simulink library "lduc_lib"  (Simulink 8.7)
settings: Solver=ode45  StartTime=0.0  StopTime=10.0  RelTol=1e-3
undefined symbols (not defined in the file): display, DUC_LINEUP_param, value
libraries: DSPBAFilters x6, DSPBAPrim x6, DSPBABase x6
settings Model: Creator=bigcat  LastModifiedBy=5g

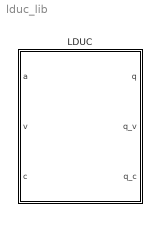
== system lduc_lib ==
  LDUC : Subsystem  mask{Clock_Margin=DUC_LINEUP_param.ClockMargin, chan_filter_SampleRate=DUC_LINEUP_param.chan_filter.SampleRate, chan_filter_ChanCount=DUC_LINEUP_param.chan_filter.ChanCount, chan_filter_coeffs=DUC_LINEUP_param.chan_filter.coeffs(1,:), chan_filter_base_addr=DUC_LINEUP_param.chan_filter.base_addr1, HB_filt4_SampleRate=DUC_LINEUP_param.HB_filt4.SampleRate, HB_filt_Interpolation=DUC_LINEUP_param.HB_filt4.Interpolation, HB_filt4_ChanCount=DUC_LINEUP_param.HB_filt4.ChanCount, HB_filt4_coeffs=DUC_LINEUP_param.HB_filt4.coeffs(1,:), HB_filt4_base_addr=DUC_LINEUP_param.HB_filt4.base_addr1, HB_filt5_SampleRate=DUC_LINEUP_param.HB_filt5.SampleRate, HB_filt5_Interpolation=DUC_LINEUP_param.HB_filt5.Interpolation, HB_filt5_ChanCount=DUC_LINEUP_param.HB_filt5.ChanCount, HB_filt5_coeffs=DUC_LINEUP_param.HB_filt5.coeffs(1,:), HB_filt5_base_addr=DUC_LINEUP_param.HB_filt5.base_addr1, Pipe_Reg=2, CH_Multiplication_fact=1, CH_Bits_to_Left_shift=0, HB4_Multiplication_fact=1, HB4_Bits_to_left_shift=1, HB5_Multiplication_fact=1, HB5_Bits_to_Left_shift=1, output_word_length=DUC_LINEUP_param.output_word_length, output_fraction_length=DUC_LINEUP_param.output_fraction_length}
      mask Display:
      | disp('LDUC');
      | port_label('input',1,'d');
      | port_label('input',2,'v');
      | port_label('input',3,'c');
      | port_label('output',1,'q');
      | port_label('output',2,'qv');
      | port_label('output',3,'qc');

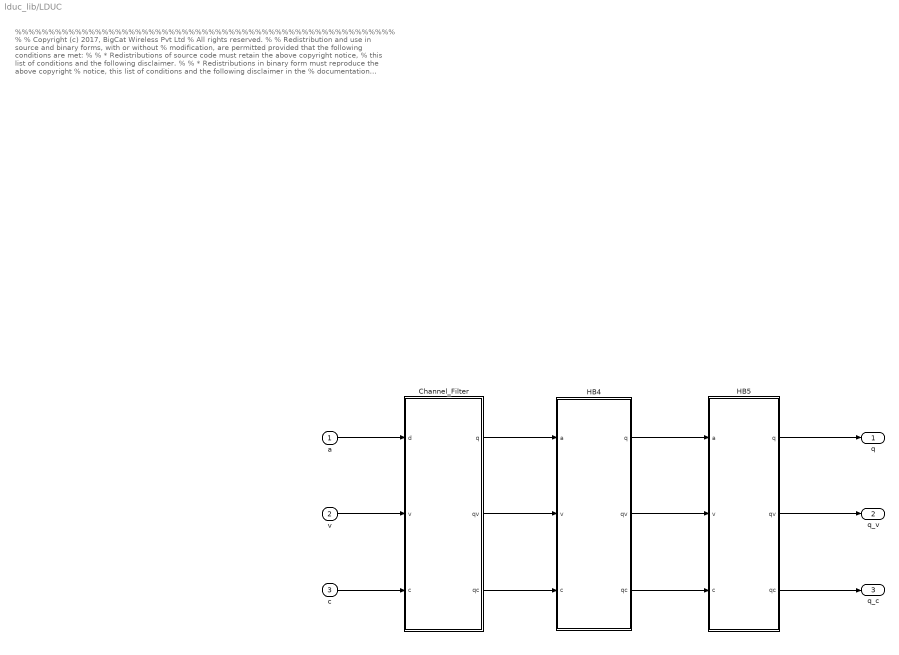
== system lduc_lib/LDUC ==
  note: %%%%%%%%%%%%%%%%%%%%%%%%%%%%%%%%%%%%%%%%%%%%%%%%%%%%%%%%%
      |  %
      |  % Copyright (c) 2017, BigCat Wireless Pvt Ltd
      |  % All rights reserved.
      |  %
      |  % Redistribution and use in source and binary forms, with or without
      |  % modification, are permitted provided that the following conditions are met:
      |  %
      |  %     * Redistributions of source code must retain the above copyright notice,
      |  %       this list of conditions and the following disclaimer.
      |  %
      |  %     * Redistributions in binary form must reproduce the above copyright
      |  %       notice, this list of conditions and the following disclaimer in the
      |  %       documentation and/or other materials provided with the distribution.
      |  %
      |  %     * Neither the name of the copyright holder nor the names of its contributors
      |  %       may be used to endorse or promote products derived from this software
      |  %       without specific prior written permission.
      |  %
      |  %
      |  %
      |  % THIS SOFTWARE IS PROVIDED BY THE COPYRIGHT HOLDERS AND CONTRIBUTORS "AS IS"
      |  % AND ANY EXPRESS OR IMPLIED WARRANTIES, INCLUDING, BUT NOT LIMITED TO, THE
      |  % IMPLIED WARRANTIES OF MERCHANTABILITY AND FITNESS FOR A PARTICULAR PURPOSE ARE
      |  % DISCLAIMED. IN NO EVENT SHALL THE COPYRIGHT HOLDER OR CONTRIBUTORS BE LIABLE
      |  % FOR ANY DIRECT, INDIRECT, INCIDENTAL, SPECIAL, EXEMPLARY, OR CONSEQUENTIAL
      |  % DAMAGES (INCLUDING, BUT NOT LIMITED TO, PROCUREMENT OF SUBSTITUTE GOODS OR
      |  % SERVICES; LOSS OF USE, DATA, OR PROFITS; OR BUSINESS INTERRUPTION) HOWEVER
      |  % CAUSED AND ON ANY THEORY OF LIABILITY, WHETHER IN CONTRACT, STRICT LIABILITY,
      |  % OR TORT (INCLUDING NEGLIGENCE OR OTHERWISE) ARISING IN ANY WAY OUT OF THE USE
      |  % OF THIS SOFTWARE, EVEN IF ADVISED OF THE POSSIBILITY OF SUCH DAMAGE.
      |  %
      |   %%%%%%%%%%%%%%%%%%%%%%%%%%%%%%%%%%%%%%%%%%%%%%%%%%%%%%%%%%
  a : Inport
  v : Inport  Port=2
  c : Inport  Port=3
  Channel_Filter : Subsystem
  HB4 : Subsystem
  HB5 : Subsystem
  q : Outport
  q_v : Outport  Port=2
  q_c : Outport  Port=3
  wires:
  Channel_Filter/3(qc) -> HB4/3(c)
  Channel_Filter/2(qv) -> HB4/2(v)
  Channel_Filter/1(q) -> HB4/1(a)
  a/1 -> Channel_Filter/1(d)
  v/1 -> Channel_Filter/2(v)
  c/1 -> Channel_Filter/3(c)
  HB5/1(q) -> q/1
  HB5/2(qv) -> q_v/1
  HB5/3(qc) -> q_c/1
  HB4/2(qv) -> HB5/2(v)
  HB4/1(q) -> HB5/1(a)
  HB4/3(qc) -> HB5/3(c)

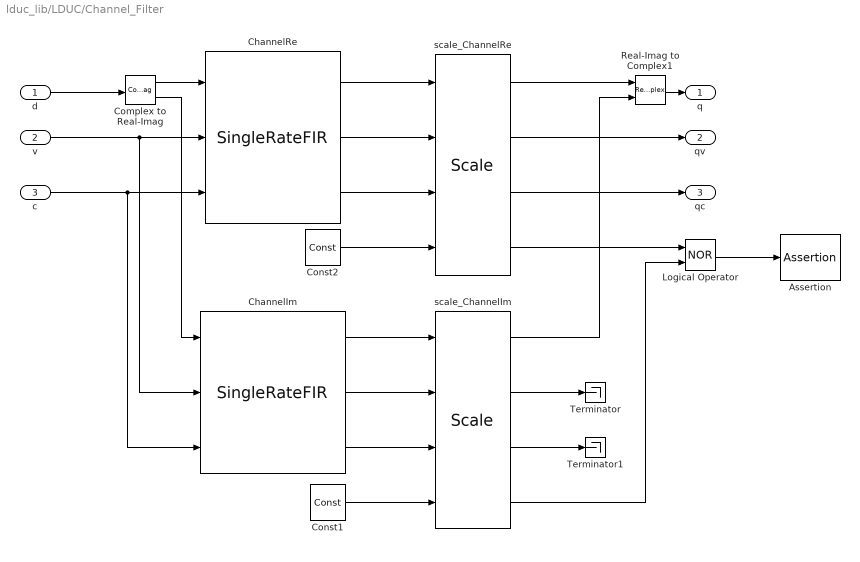
== system lduc_lib/LDUC/Channel_Filter ==
  d : Inport
  v : Inport  Port=2
  c : Inport  Port=3
  Assertion : Assertion  Enabled=off  AssertionFailFcn=display('Simulation stopped because of over/underflow in channel filter in LDUC')
  ChannelIm : DSPBAFilters/SingleRateFIR  nInputRate=chan_filter_SampleRate  nchan=chan_filter_ChanCount/2  symmetry=Symmetrical  coef=chan_filter_coeffs(1,:)  addr=chan_filter_base_addr+128  rwmode=Read/Write  nband=Use All Taps  latency=4  exposebus=off  version=20090407  recon=off  MM=[0,1,2,3,4,5,6,7,8,9,10,11,12,13,14,15;0,1,2,3,4,5,6,7,8,9,10,11,12,13,14,15]
  ChannelRe : DSPBAFilters/SingleRateFIR  nInputRate=chan_filter_SampleRate  nchan=chan_filter_ChanCount/2  symmetry=Symmetrical  coef=chan_filter_coeffs(1,:)  addr=chan_filter_base_addr  rwmode=Read/Write  nband=Use All Taps  latency=4  exposebus=off  version=20090407  recon=off  MM=[0,1,2,3,4,5,6,7,8,9,10,11,12,13,14,15;0,1,2,3,4,5,6,7,8,9,10,11,12,13,14,15]
  Complex to Real-Imag : ComplexToRealImag
  Const1 : DSPBAPrim/Const  primtype=const  nInputs=0  nOutputs=1  omode=Inherit via internal rule  otype=sfix(16)  scale=2^-15  rndmethod=Unbiased  factor=1  satmethod=Symmetric  shift_vec=[0 1 2 -1]  value=0  inPortNames=['+'; '+';]  outPortNames=[' ']  dspbaimage=dspba_prim.jpg  text=fprintf('%s', num2str(value));  style=Optimised  visibilities=8 + 1024  floatPrecision=float32_m23  version=20120820
  Const2 : DSPBAPrim/Const  primtype=const  nInputs=0  nOutputs=1  omode=Inherit via internal rule  otype=sfix(16)  scale=2^-15  rndmethod=Unbiased  factor=1  satmethod=Symmetric  shift_vec=[0 1 2 -1]  value=0  inPortNames=['+'; '+';]  outPortNames=[' ']  dspbaimage=dspba_prim.jpg  text=fprintf('%s', num2str(value));  style=Optimised  visibilities=8 + 1024  floatPrecision=float32_m23  version=20120820
  Logical Operator : Logic  Operator=NOR  AllPortsSameDT=off  OutDataTypeStr=boolean
  Real-Imag to Complex1 : RealImagToComplex
  Terminator : Terminator
  Terminator1 : Terminator
  scale_ChannelIm : DSPBABase/Scale  otype=sfix(output_word_length)  scale=2^-output_fraction_length  rndmethod=Truncate  factor=CH_Multiplication_fact  satmethod=Symmetric  shift_vec=CH_Bits_to_Left_shift  latency=4  wideSimulation=off  version=20090407
  scale_ChannelRe : DSPBABase/Scale  otype=sfix(output_word_length)  scale=2^-output_fraction_length  rndmethod=Truncate  factor=CH_Multiplication_fact  satmethod=Symmetric  shift_vec=CH_Bits_to_Left_shift  latency=4  wideSimulation=off  version=20090407
  q : Outport
  qv : Outport  Port=2
  qc : Outport  Port=3
  wires:
  Logical Operator/1 -> Assertion/1
  scale_ChannelIm/4 -> Logical Operator/2
  scale_ChannelIm/3 -> Terminator1/1
  scale_ChannelIm/2 -> Terminator/1
  scale_ChannelIm/1 -> Real-Imag to Complex1/2
  ChannelIm/3 -> scale_ChannelIm/3
  ChannelIm/2 -> scale_ChannelIm/2
  ChannelIm/1 -> scale_ChannelIm/1
  Real-Imag to Complex1/1 -> q/1
  scale_ChannelRe/1 -> Real-Imag to Complex1/1
  Const1/1 -> scale_ChannelIm/4
  Complex to Real-Imag/2 -> ChannelIm/1
  Complex to Real-Imag/1 -> ChannelRe/1
  d/1 -> Complex to Real-Imag/1
  ChannelRe/1 -> scale_ChannelRe/1
  c/1 -> ChannelIm/3, ChannelRe/3
  v/1 -> ChannelIm/2, ChannelRe/2
  scale_ChannelRe/3 -> qc/1
  Const2/1 -> scale_ChannelRe/4
  scale_ChannelRe/2 -> qv/1
  ChannelRe/2 -> scale_ChannelRe/2
  ChannelRe/3 -> scale_ChannelRe/3
  scale_ChannelRe/4 -> Logical Operator/1

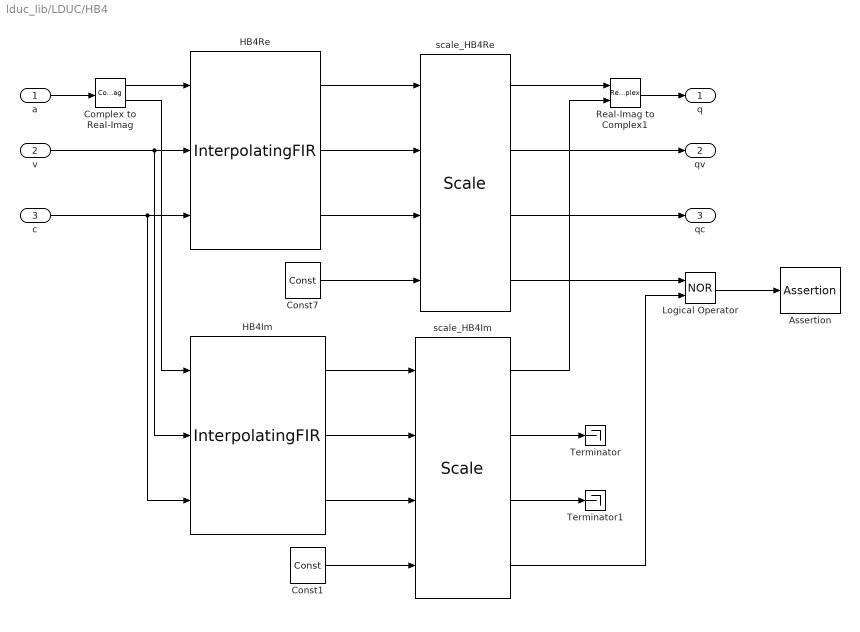
== system lduc_lib/LDUC/HB4 ==
  a : Inport
  v : Inport  Port=2
  c : Inport  Port=3
  Assertion : Assertion  Enabled=off  AssertionFailFcn=display('Simulation stopped because of over/underflow in HB4 filter in LDUC')
  Complex to Real-Imag : ComplexToRealImag
  Const1 : DSPBAPrim/Const  primtype=const  nInputs=0  nOutputs=1  omode=Inherit via internal rule  otype=sfix(16)  scale=2^-15  rndmethod=Unbiased  factor=1  satmethod=Symmetric  shift_vec=[0 1 2 -1]  value=0  inPortNames=['+'; '+';]  outPortNames=[' ']  dspbaimage=dspba_prim.jpg  text=fprintf('%s', num2str(value));  style=Optimised  visibilities=8 + 1024  floatPrecision=float32_m23  version=20120820
  Const7 : DSPBAPrim/Const  primtype=const  nInputs=0  nOutputs=1  omode=Inherit via internal rule  otype=sfix(16)  scale=2^-15  rndmethod=Unbiased  factor=1  satmethod=Symmetric  shift_vec=[0 1 2 -1]  value=0  inPortNames=['+'; '+';]  outPortNames=[' ']  dspbaimage=dspba_prim.jpg  text=fprintf('%s', num2str(value));  style=Optimised  visibilities=8 + 1024  floatPrecision=float32_m23  version=20120820
  HB4Im : DSPBAFilters/InterpolatingFIR  nInputRate=HB_filt4_SampleRate  interp=HB_filt_Interpolation  nchan=HB_filt4_ChanCount/2  symmetry=Symmetrical  coef=HB_filt4_coeffs(1,:)  addr=HB_filt4_base_addr+128  rwmode=Constant  nband=Half Band  exposebus=off  latency=14  version=20090407  recon=off  MM=[0,1,2,3,4,5,6,7,8,9,10,11,12,13,14,15]
  HB4Re : DSPBAFilters/InterpolatingFIR  nInputRate=HB_filt4_SampleRate  interp=HB_filt_Interpolation  nchan=HB_filt4_ChanCount/2  symmetry=Symmetrical  coef=HB_filt4_coeffs(1,:)  addr=HB_filt4_base_addr  rwmode=Constant  nband=Half Band  exposebus=off  latency=14  version=20090407  recon=off  MM=[0,1,2,3,4,5,6,7,8,9,10,11,12,13,14,15]
  Logical Operator : Logic  Operator=NOR  AllPortsSameDT=off  OutDataTypeStr=boolean
  Real-Imag to Complex1 : RealImagToComplex
  Terminator : Terminator
  Terminator1 : Terminator
  scale_HB4Im : DSPBABase/Scale  otype=sfix(output_word_length)  scale=2^-output_fraction_length  rndmethod=Truncate  factor=HB4_Multiplication_fact  satmethod=Symmetric  shift_vec=HB4_Bits_to_left_shift  latency=4  wideSimulation=off  version=20090407
  scale_HB4Re : DSPBABase/Scale  otype=sfix(output_word_length)  scale=2^-output_fraction_length  rndmethod=Truncate  factor=HB4_Multiplication_fact  satmethod=Symmetric  shift_vec=HB4_Bits_to_left_shift  latency=4  wideSimulation=off  version=20090407
  q : Outport
  qv : Outport  Port=2
  qc : Outport  Port=3
  wires:
  Logical Operator/1 -> Assertion/1
  scale_HB4Im/4 -> Logical Operator/2
  scale_HB4Im/3 -> Terminator1/1
  scale_HB4Im/2 -> Terminator/1
  Real-Imag to Complex1/1 -> q/1
  scale_HB4Im/1 -> Real-Imag to Complex1/2
  HB4Im/3 -> scale_HB4Im/3
  HB4Im/2 -> scale_HB4Im/2
  scale_HB4Re/1 -> Real-Imag to Complex1/1
  Const1/1 -> scale_HB4Im/4
  HB4Im/1 -> scale_HB4Im/1
  Complex to Real-Imag/2 -> HB4Im/1
  HB4Re/1 -> scale_HB4Re/1
  Complex to Real-Imag/1 -> HB4Re/1
  a/1 -> Complex to Real-Imag/1
  Const7/1 -> scale_HB4Re/4
  HB4Re/3 -> scale_HB4Re/3
  HB4Re/2 -> scale_HB4Re/2
  scale_HB4Re/3 -> qc/1
  scale_HB4Re/2 -> qv/1
  scale_HB4Re/4 -> Logical Operator/1
  c/1 -> HB4Im/3, HB4Re/3
  v/1 -> HB4Im/2, HB4Re/2

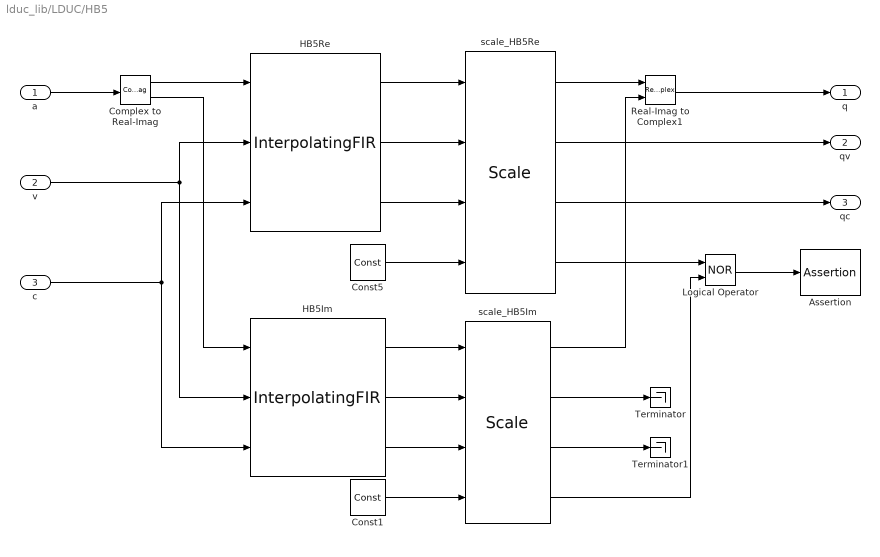
== system lduc_lib/LDUC/HB5 ==
  a : Inport
  v : Inport  Port=2
  c : Inport  Port=3
  Assertion : Assertion  Enabled=off  AssertionFailFcn=display('Simulation stopped because of over/underflow in HB4 filter in LDUC')
  Complex to Real-Imag : ComplexToRealImag
  Const1 : DSPBAPrim/Const  primtype=const  nInputs=0  nOutputs=1  omode=Inherit via internal rule  otype=sfix(16)  scale=2^-15  rndmethod=Unbiased  factor=1  satmethod=Symmetric  shift_vec=[0 1 2 -1]  value=0  inPortNames=['+'; '+';]  outPortNames=[' ']  dspbaimage=dspba_prim.jpg  text=fprintf('%s', num2str(value));  style=Optimised  visibilities=8 + 1024  floatPrecision=float32_m23  version=20120820
  Const5 : DSPBAPrim/Const  primtype=const  nInputs=0  nOutputs=1  omode=Inherit via internal rule  otype=sfix(16)  scale=2^-15  rndmethod=Unbiased  factor=1  satmethod=Symmetric  shift_vec=[0 1 2 -1]  value=0  inPortNames=['+'; '+';]  outPortNames=[' ']  dspbaimage=dspba_prim.jpg  text=fprintf('%s', num2str(value));  style=Optimised  visibilities=8 + 1024  floatPrecision=float32_m23  version=20120820
  HB5Im : DSPBAFilters/InterpolatingFIR  nInputRate=HB_filt5_SampleRate  interp=HB_filt5_Interpolation  nchan=HB_filt5_ChanCount/2  symmetry=Symmetrical  coef=HB_filt5_coeffs(1,:)  addr=HB_filt5_base_addr+128  rwmode=Constant  nband=Half Band  exposebus=off  latency=10  version=20090407  recon=off  MM=[0,1,2,3,4,5,6,7,8,9,10,11,12,13,14,15]
  HB5Re : DSPBAFilters/InterpolatingFIR  nInputRate=HB_filt5_SampleRate  interp=HB_filt5_Interpolation  nchan=HB_filt5_ChanCount/2  symmetry=Symmetrical  coef=HB_filt5_coeffs(1,:)  addr=HB_filt5_base_addr  rwmode=Constant  nband=Half Band  exposebus=off  latency=10  version=20090407  recon=off  MM=[0,1,2,3,4,5,6,7,8,9,10,11,12,13,14,15]
  Logical Operator : Logic  Operator=NOR  AllPortsSameDT=off  OutDataTypeStr=boolean
  Real-Imag to Complex1 : RealImagToComplex
  Terminator : Terminator
  Terminator1 : Terminator
  scale_HB5Im : DSPBABase/Scale  otype=sfix(output_word_length)  scale=2^-output_fraction_length  rndmethod=Truncate  factor=HB5_Multiplication_fact  satmethod=Symmetric  shift_vec=HB5_Bits_to_Left_shift  latency=4  wideSimulation=off  version=20090407
  scale_HB5Re : DSPBABase/Scale  otype=sfix(output_word_length)  scale=2^-output_fraction_length  rndmethod=Truncate  factor=HB5_Multiplication_fact  satmethod=Symmetric  shift_vec=HB5_Bits_to_Left_shift  latency=4  wideSimulation=off  version=20090407
  q : Outport
  qv : Outport  Port=2
  qc : Outport  Port=3
  wires:
  Logical Operator/1 -> Assertion/1
  scale_HB5Im/4 -> Logical Operator/2
  scale_HB5Im/3 -> Terminator1/1
  scale_HB5Im/2 -> Terminator/1
  scale_HB5Im/1 -> Real-Imag to Complex1/2
  HB5Im/3 -> scale_HB5Im/3
  HB5Im/2 -> scale_HB5Im/2
  HB5Im/1 -> scale_HB5Im/1
  scale_HB5Re/1 -> Real-Imag to Complex1/1
  Real-Imag to Complex1/1 -> q/1
  Const1/1 -> scale_HB5Im/4
  c/1 -> HB5Re/3, HB5Im/3
  Complex to Real-Imag/2 -> HB5Im/1
  HB5Re/1 -> scale_HB5Re/1
  Complex to Real-Imag/1 -> HB5Re/1
  a/1 -> Complex to Real-Imag/1
  scale_HB5Re/3 -> qc/1
  HB5Re/3 -> scale_HB5Re/3
  HB5Re/2 -> scale_HB5Re/2
  scale_HB5Re/2 -> qv/1
  Const5/1 -> scale_HB5Re/4
  scale_HB5Re/4 -> Logical Operator/1
  v/1 -> HB5Re/2, HB5Im/2
